simulink model "ES249B_MotAgCorrln"  (R2013b)
settings: Solver=FixedStepDiscrete  SolverMode=SingleTasking  StartTime=0.0  StopTime=1  FixedStep=0.002  RelTol=1e-3
values from neighbouring files (symbols this model uses):
  FLTINJ_MOTAGCORRLN_MOTAGIDPTSIG = DataDict.Constant    [ES249B_MotAgCorrln_DataDict.m]
  HALFREV_MOTREV_U0P16 = DataDict.Constant    [ES249B_MotAgCorrln_DataDict.m]
  MOTAGACORRLNST_CNT_U08 = DataDict.Constant    [ES249B_MotAgCorrln_DataDict.m]
  MotAgAMotAgBCorrln = DataDict.NTC    [ES249B_MotAgCorrln_DataDict.m]
  MOTAGBCORRLNST_CNT_U08 = DataDict.Constant    [ES249B_MotAgCorrln_DataDict.m]
  MOTAGCORRLNERRTHD_MOTREVELEC_U0P16 = DataDict.Constant    [ES249B_MotAgCorrln_DataDict.m]
  MOTAGCORRLNNTCFAILSTEP_CNT_U16 = DataDict.Constant    [ES249B_MotAgCorrln_DataDict.m]
  MOTAGCORRLNNTCPASSSTEP_CNT_U16 = DataDict.Constant    [ES249B_MotAgCorrln_DataDict.m]
  MOTAGMAXSTALLCNTR_CNT_U08 = DataDict.Constant    [ES249B_MotAgCorrln_DataDict.m]
  MotAgMeclCorrlnSt = DataDict.OpSignal    [ES249B_MotAgCorrln_DataDict.m]
  MotAgMeclIdptSig = DataDict.OpSignal    [ES249B_MotAgCorrln_DataDict.m]
  SysGlbPrmMotPoleCnt = DataDict.ImprtdCal    [ES249B_MotAgCorrln_DataDict.m]
undefined symbols (not defined in the file or in its folder): NtcSts1, sigbuilder_block, SigQlfr1
libraries: simulink x5
(part 1 of 2)
settings Model: Creator=pz79n7  LastModifiedBy=FZG88Y
settings SolverCC: AutoInsertRateTranBlk=on  InsertRTBMode=Always
settings DataIOCC: LimitDataPoints=off  SaveFormat=Structure  ReturnWorkspaceOutputs=on
settings OptimizationCC: BlockReduction=off  InlineParams=on  ZeroExternalMemoryAtStartup=off  ZeroInternalMemoryAtStartup=off  OptimizeModelRefInitCode=on  LifeSpan=1
settings DebuggingCC: SignalInfNanChecking=error  SignalRangeChecking=warning  UnderspecifiedInitializationDetection=Simplified  SolverPrmCheckMsg=error  InheritedTsInSrcMsg=error  DiscreteInheritContinuousMsg=error  SingleTaskRateTransMsg=error  TasksWithSamePriorityMsg=error  SigSpecEnsureSampleTimeMsg=error  CheckMatrixSingularityMsg=error  ParameterUnderflowMsg=error  ParameterPrecisionLossMsg=error  ParameterTunabilityLossMsg=error  FixptConstUnderflowMsg=warning  FixptConstOverflowMsg=warning  VectorMatrixConversionMsg=error  SignalLabelMismatchMsg=error  UnconnectedInputMsg=error  UnconnectedOutputMsg=error  UnconnectedLineMsg=error  SFcnCompatibilityMsg=error  UniqueDataStoreMsg=warning  BusObjectLabelMismatch=error  RootOutportRequireBusObject=error  AssertControl=DisableAll  ModelReferenceIOMsg=error  ModelReferenceVersionMismatchMessage=warning  ModelReferenceIOMismatchMessage=error  ModelReferenceCSMismatchMessage=warning  ModelReferenceDataLoggingMessage=error  StateNameClashWarn=warning  StrictBusMsg=ErrorOnBusTreatedAsVector  NonBusSignalsTreatedAsBus=error  SFUnexpectedBacktrackingDiag=error  SFInvalidInputDataAccessInChartInitDiag=error  SFNoUnconditionalDefaultTransitionDiag=error  SFTransitionOutsideNaturalParentDiag=error  SFUnconditionalTransitionShadowingDiag=error  SFUndirectedBroadcastEventsDiag=error
settings ModelReferenceCC: ModelReferenceNumInstancesAllowed=Single
settings RTWCC: SystemTargetFile=autosar.tlc  GenCodeOnly=on  TemplateMakefile=ert_default_tmf  Description=AUTOSAR  GenerateReport=on  ProcessScript=autosar_make_rtw_hook  LaunchReport=on
settings CodeAppCC: GenerateComments=off  IgnoreCustomStorageClasses=off  CustomSymbolStrType=$N$R$M  CustomSymbolStrBlkIO=$N$M  SimulinkBlockComments=off
settings STFCustomTargetCC: ParMdlRefBuildCompliant=on  CompOptLevelCompliant=on  IncludeMdlTerminateFcn=off  CombineOutputUpdateFcns=on  SuppressErrorStatus=on  ERTFirstTimeCompliant=on  ERTCustomFileBanners=on  SupportNonFinite=off  SupportComplex=off  SupportContinuousTime=off  SupportNonInlinedSFcns=off  MATLABClassNameForMDSCustomization=Simulink.SoftwareTarget.ERTCustomization  AutosarCompliant=on  GRTInterface=off  SystemTargetFile=autosar.tlc
settings ERTTargetCC: CodeReplacementLibrary=ANSI_C  ConcurrentExecutionCompliant=off  IncludeMdlTerminateFcn=off  SuppressErrorStatus=on  SupportNonFinite=off  SupportComplex=off  ModelStepFunctionPrototypeControlCompliant=off  CPPClassGenCompliant=off  AutosarCompliant=on  InlinedParameterPlacement=NonHierarchical  ERTCustomFileTemplate=example_file_process.tlc  EnableUserReplacementTypes=on

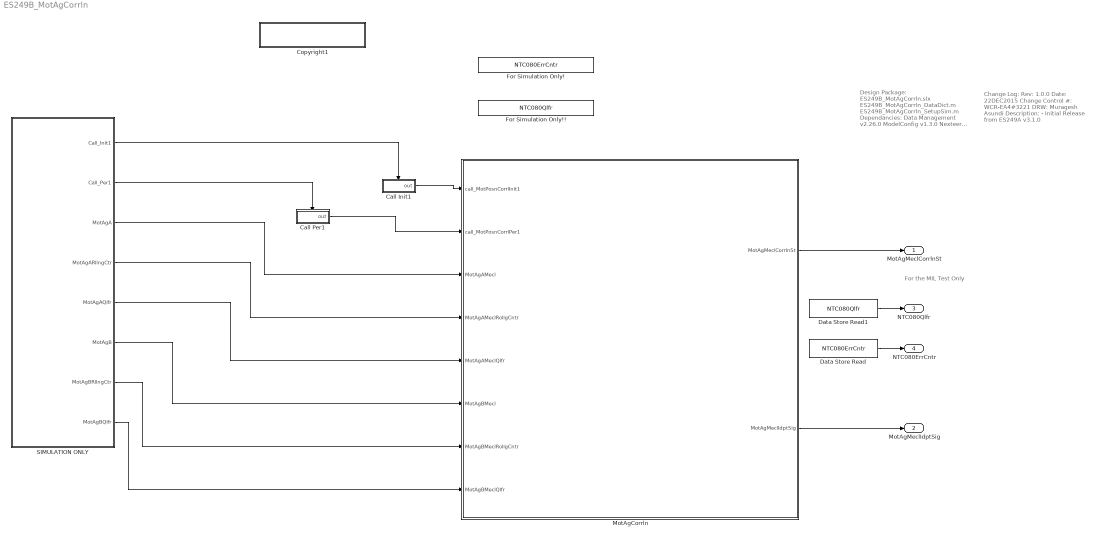
== system ES249B_MotAgCorrln ==
  note: Change Log:
      |
      | Rev: 1.0.0
      | Date: 22DEC2015
      | Change Control #: WCR-EA4#3221
      | DRW: Muragesh Asundi
      | Description:
      | - Initial Release from ES249A v3.1.0
  note: Design Package:
      | ES249B_MotAgCorrln.slx
      | ES249B_MotAgCorrln_DataDict.m
      | ES249B_MotAgCorrln_SetupSim.m
      |
      | Dependancies:
      |    Data Management v2.26.0
      |    ModelConfig v1.3.0
      |    Nexteer Utilities v4.5.0
      |    Tools v1.9.0
      |
      | Requirement: 1.0
  note: For the MIL Test Only
  Call Init1 : Subsystem  TreatAsAtomicUnit=on
  Call Per1 : Subsystem  TreatAsAtomicUnit=on
  Copyright1 : Subsystem  Description=|  mask(Copyright Information){none=on}
      | Copyright info block.                                               
      |                                                                     
      | Place copyright information at the top of every subsystem in design.
      mask prompts: none "No parameters"
      mask help: Place copyright information at the top of every subsystem in design.
      mask Display:
      | NxtrConf = 'Nexteer Confidential';
      | 
      | sys = bdroot; %handle for the current model ("system")
      | first = get_param(sys,'Created');
      | if(isempty(first))
      |     first = datestr(now,'yyyy');
      | else
      |     first = first(end-3:end);  %year is last four digits
      | end
      | 
      | last = get_param(sys,'LastModifiedDate');
      | if isempty(last)
      |     last = datestr(now,'yyyy');
      | else
      |     last = last(end-3:end);
      | end
      | 
      | if strcmp(first,last)
      |     fprintf('%s\nCopyright  %s Nexteer',NxtrConf,first);
      | else
      |     fprintf('%s\n%s%s-%s Nexteer',NxtrConf,char(169),first,last);
      | end
  Data Store Read : DataStoreRead  DataStoreName=NTC080ErrCntr  SampleTime=0.002
  Data Store Read1 : DataStoreRead  DataStoreName=NTC080Qlfr  SampleTime=0.002
  For Simulation Only! : DataStoreMemory  DataStoreName=NTC080ErrCntr
  For Simulation Only!! : DataStoreMemory  DataStoreName=NTC080Qlfr
  MotAgCorrln : Subsystem
  SIMULATION ONLY : Subsystem
  MotAgMeclCorrlnSt : Outport  RequirementInfo={} %GIDa_d8739ec6_a18f_4415_a443_47ea44f287a3
  MotAgMeclIdptSig : Outport  RequirementInfo={} %GIDa_85b325d8_f6bf_41e3_b16b_50e782c8add7  Port=2
  NTC080Qlfr : Outport  RequirementInfo={} %GIDa_3e943792_cbbb_4e5d_9230_63e142ecdc6f  Port=3
  NTC080ErrCntr : Outport  RequirementInfo={} %GIDa_f9c3ca75_2980_486f_8311_d7072cc6ecd3  Port=4
  wires:
  Call Per1/1(out) -> MotAgCorrln/2(call_MotPosnCorrlPer1)
  MotAgCorrln/1(MotAgMeclCorrlnSt) -> MotAgMeclCorrlnSt/1
  MotAgCorrln/2(MotAgMeclIdptSig) -> MotAgMeclIdptSig/1
  SIMULATION ONLY/3(MotAgA) -> MotAgCorrln/3(MotAgAMecl)
  SIMULATION ONLY/4(MotAgARllngCtr) -> MotAgCorrln/4(MotAgAMeclRollgCntr)
  SIMULATION ONLY/5(MotAgAQlfr) -> MotAgCorrln/5(MotAgAMeclQlfr)
  Call Init1/1(out) -> MotAgCorrln/1(call_MotPosnCorrlInit1)
  SIMULATION ONLY/1(Call_Init1) -> Call Init1/Enable
  SIMULATION ONLY/2(Call_Per1) -> Call Per1/Enable
  SIMULATION ONLY/8(MotAgBQlfr) -> MotAgCorrln/8(MotAgBMeclQlfr)
  SIMULATION ONLY/6(MotAgB) -> MotAgCorrln/6(MotAgBMecl)
  SIMULATION ONLY/7(MotAgBRllngCtr) -> MotAgCorrln/7(MotAgBMeclRollgCntr)
  Data Store Read1/1 -> NTC080Qlfr/1
  Data Store Read/1 -> NTC080ErrCntr/1

== system ES249B_MotAgCorrln/Call Init1 ==
  Enable : EnablePort
  Function Call Trigger : simulink/Ports & Subsystems/Function-Call Generator  RequirementInfo={} %GIDa_ff755a2e_49d1_45f7_8591_3ce0ef475338  sample_time=0  numberOfIterations=1
  out : Outport
  wires:
  Function Call Trigger/1 -> out/1

== system ES249B_MotAgCorrln/Call Per1 ==
  Enable : EnablePort
  Function Call Trigger : simulink/Ports & Subsystems/Function-Call Generator  RequirementInfo={} %GIDa_c055ea22_668e_465c_aa17_4b0a8dd99bf7  sample_time=0.002  numberOfIterations=1
  out : Outport
  wires:
  Function Call Trigger/1 -> out/1

== system ES249B_MotAgCorrln/Copyright1 ==

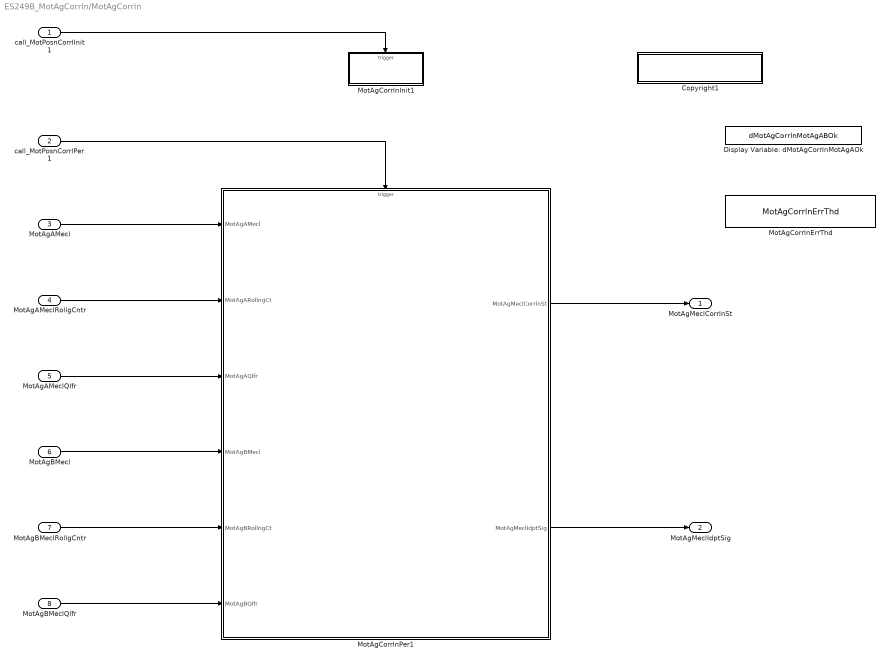
== system ES249B_MotAgCorrln/MotAgCorrln ==
  call_MotPosnCorrlInit1 : Inport  RequirementInfo={} %GIDa_df7b2033_8a98_4878_957d_25acf0131f4b
  call_MotPosnCorrlPer1 : Inport  RequirementInfo={} %GIDa_1551d67e_f818_426a_9cf4_9f4ba82b3f43  Port=2
  MotAgAMecl : Inport  RequirementInfo={'linktype_rmi_doors' '0000cf69 (/E-STEER Core/SubSystem Specifications/Electrical Actuator/Control Module/FDD Module Requirements/EA4/ES249B_MotAgCorrln)' '#ES249B_48' 'true' 'REQ: ES249B_48' '' } %GIDa_ab802314_3944_43a8_9f34_099947b7f787  Port=3
  MotAgAMeclRollgCntr : Inport  RequirementInfo={'linktype_rmi_doors' '0000cf69 (/E-STEER Core/SubSystem Specifications/Electrical Actuator/Control Module/FDD Module Requirements/EA4/ES249B_MotAgCorrln)' '#ES249B_49' 'true' 'REQ: ES249B_49' '' } %GIDa_a38bab73_f7bf_4755_8745_3afc46561306  Port=4
  MotAgAMeclQlfr : Inport  RequirementInfo={'linktype_rmi_doors' '0000cf69 (/E-STEER Core/SubSystem Specifications/Electrical Actuator/Control Module/FDD Module Requirements/EA4/ES249B_MotAgCorrln)' '#ES249B_65' 'true' 'REQ: ES249B_65' '' } %GIDa_033694cf_56a5_4107_96d0_836401cb9721  Port=5
  MotAgBMecl : Inport  RequirementInfo={'linktype_rmi_doors' '0000cf69 (/E-STEER Core/SubSystem Specifications/Electrical Actuator/Control Module/FDD Module Requirements/EA4/ES249B_MotAgCorrln)' '#ES249B_66' 'true' 'REQ: ES249B_66' '' } %GIDa_ed21c9ba_4edb_4b2f_a77a_49cd20ecbf68  Port=6
  MotAgBMeclRollgCntr : Inport  RequirementInfo={'linktype_rmi_doors' '0000cf69 (/E-STEER Core/SubSystem Specifications/Electrical Actuator/Control Module/FDD Module Requirements/EA4/ES249B_MotAgCorrln)' '#ES249B_67' 'true' 'REQ: ES249B_67' '' } %GIDa_6e6bb4b4_2d5c_4f1b_b4e7_5884c06a9259  Port=7
  MotAgBMeclQlfr : Inport  RequirementInfo={'linktype_rmi_doors' '0000cf69 (/E-STEER Core/SubSystem Specifications/Electrical Actuator/Control Module/FDD Module Requirements/EA4/ES249B_MotAgCorrln)' '#ES249B_68' 'true' 'REQ: ES249B_68' '' } %GIDa_842dc15f_0b28_4c0e_80ed_768af48a7cab  Port=8
  Copyright1 : Subsystem  Description=|  RequirementInfo={} %GIDa_dd7bc4e6_4adb_4397_9a47_107977c533a5  mask(Copyright Information){none=on}
      | Copyright info block.                                               
      |                                                                     
      | Place copyright information at the top of every subsystem in design.
      mask prompts: none "No parameters"
      mask help: Place copyright information at the top of every subsystem in design.
      mask Display:
      | NxtrConf = 'Nexteer Confidential';
      | 
      | sys = bdroot; %handle for the current model ("system")
      | first = get_param(sys,'Created');
      | if(isempty(first))
      |     first = datestr(now,'yyyy');
      | else
      |     first = first(end-3:end);  %year is last four digits
      | end
      | 
      | last = get_param(sys,'LastModifiedDate');
      | if isempty(last)
      |     last = datestr(now,'yyyy');
      | else
      |     last = last(end-3:end);
      | end
      | 
      | if strcmp(first,last)
      |     fprintf('%s\nCopyright  %s Nexteer',NxtrConf,first);
      | else
      |     fprintf('%s\n%s%s-%s Nexteer',NxtrConf,char(169),first,last);
      | end
  Display Variable: dMotAgCorrlnMotAgAOk : DataStoreMemory  DataStoreName=dMotAgCorrlnMotAgABOk  StateMustResolveToSignalObject=on
  MotAgCorrlnErrThd : DataStoreMemory  Priority=0  DataStoreName=MotAgCorrlnErrThd  StateMustResolveToSignalObject=on
  MotAgCorrlnInit1 : Subsystem  TreatAsAtomicUnit=on
  MotAgCorrlnPer1 : Subsystem  RequirementInfo={} %GIDa_e8c7526b_9849_4008_8b1a_56f97ffa1c8d  TreatAsAtomicUnit=on
  MotAgMeclCorrlnSt : Outport  RequirementInfo={'linktype_rmi_doors' '0000cf69 (/E-STEER Core/SubSystem Specifications/Electrical Actuator/Control Module/FDD Module Requirements/EA4/ES249B_MotAgCorrln)' '#ES249B_51' 'true' 'REQ: ES249B_51' '' } %GIDa_ae509c2f_e3de_4035_9028_020cbec86e82
  MotAgMeclIdptSig : Outport  RequirementInfo={'linktype_rmi_doors' '0000cf69 (/E-STEER Core/SubSystem Specifications/Electrical Actuator/Control Module/FDD Module Requirements/EA4/ES249B_MotAgCorrln)' '#ES249B_52' 'true' 'REQ: ES249B_52' '' } %GIDa_df68f2b0_a0f0_444f_88a1_35645a7edbac  Port=2
  wires:
  call_MotPosnCorrlPer1/1 -> MotAgCorrlnPer1/Trigger
  MotAgCorrlnPer1/2(MotAgMeclIdptSig) -> MotAgMeclIdptSig/1
  MotAgCorrlnPer1/1(MotAgMeclCorrlnSt) -> MotAgMeclCorrlnSt/1
  MotAgAMecl/1 -> MotAgCorrlnPer1/1(MotAgAMecl)
  MotAgAMeclRollgCntr/1 -> MotAgCorrlnPer1/2(MotAgARollngCt)
  MotAgAMeclQlfr/1 -> MotAgCorrlnPer1/3(MotAgAQlfr)
  MotAgBMecl/1 -> MotAgCorrlnPer1/4(MotAgBMecl)
  MotAgBMeclRollgCntr/1 -> MotAgCorrlnPer1/5(MotAgBRollngCt)
  MotAgBMeclQlfr/1 -> MotAgCorrlnPer1/6(MotAgBQlfr)
  call_MotPosnCorrlInit1/1 -> MotAgCorrlnInit1/Trigger

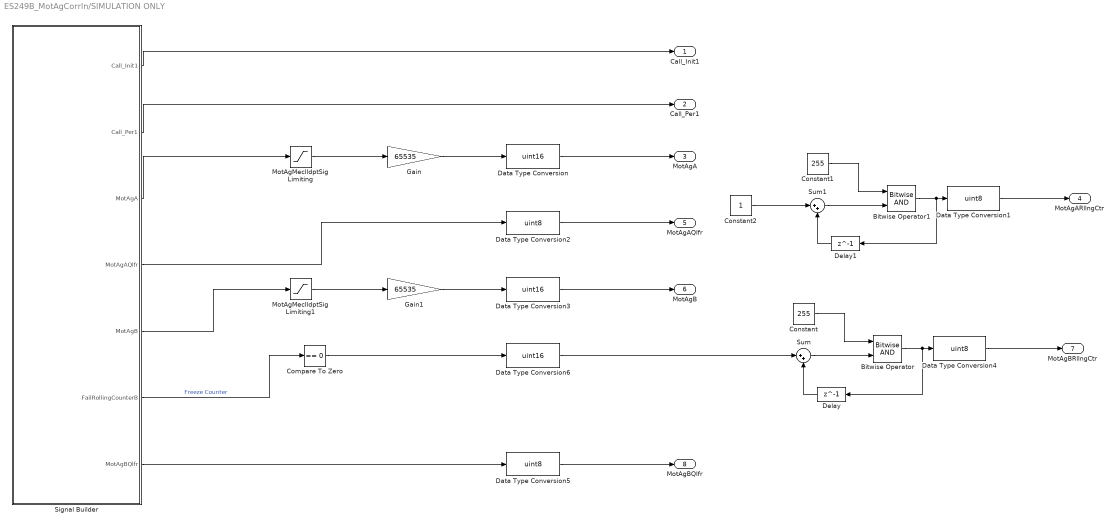
== system ES249B_MotAgCorrln/SIMULATION ONLY ==
  Bitwise Operator : simulink/Logic and Bit Operations/Bitwise Operator  logicop=AND  UseBitMask=off  NumInputPorts=2  BitMask=bin2dec('11011001')  BitMaskRealWorld=Stored Integer
  Bitwise Operator1 : simulink/Logic and Bit Operations/Bitwise Operator  logicop=AND  UseBitMask=off  NumInputPorts=2  BitMask=bin2dec('11011001')  BitMaskRealWorld=Stored Integer
  Compare To Zero : simulink/Logic and Bit Operations/Compare To Zero  relop===  OutDataTypeStr=boolean
  Constant : Constant  Value=255  OutDataTypeStr=uint16
  Constant1 : Constant  Value=255  OutDataTypeStr=uint16
  Constant2 : Constant  OutDataTypeStr=uint16
  Data Type Conversion : DataTypeConversion  OutDataTypeStr=uint16
  Data Type Conversion{1..2,4..5} (4 alike) : DataTypeConversion  OutDataTypeStr=uint8
  Data Type Conversion3 : DataTypeConversion  OutDataTypeStr=uint16
  Data Type Conversion6 : DataTypeConversion  OutDataTypeStr=uint16
  Delay : Delay  DelayLength=1  InitialCondition=0  SampleTime=0.002
  Delay1 : Delay  DelayLength=1  InitialCondition=0  SampleTime=0.002
  Gain : Gain  Gain=65535
  Gain1 : Gain  Gain=65535
  MotAgMeclIdptSig Limiting : Saturate  UpperLimit=1  LowerLimit=0
  MotAgMeclIdptSig Limiting1 : Saturate  UpperLimit=MotAgMeclIdptSig.EngMax  LowerLimit=MotAgMeclIdptSig.EngMin
  Signal Builder : Subsystem  Tag=STV Subsys  LoadFcn=sigbuilder_block('load');  StartFcn=sigbuilder_block('start');  StopFcn=sigbuilder_block('stop');  ClipboardFcn=sigbuilder_block('clipboard');  mask(Sigbuilder block){}
      mask help: Simulink:masks:SigbuilderBlock_MD
      mask init:
      | if ~strcmp(get_param(bdroot(gcbh),'SimulationStatus'),'stopped') tuvar = sigbuilder_block('maskInit'); end
      settings: CopyFcn=sigbuilder_block('copy');  DeleteFcn=sigbuilder_block('delete');  ModelCloseFcn=sigbuilder_block('modelClose');  PreSaveFcn=sigbuilder_block('preSave');  PauseFcn=sigbuilder_block('pause');  ContinueFcn=sigbuilder_block('continue');  NameChangeFcn=sigbuilder_block('namechange');  OpenFcn=sigbuilder_block('open',[6 6 1012.5 507 ]);  CloseFcn=sigbuilder_block('close');
      mask Display: plot(0, 0, 100, 100,[2, 2, 32, 32, 2], [68, 8, 8, 68, 68],[32, 2], [38, 38], [32, 19, 2],[53, 60, 44], [32, 17, 17, 2],[16, 16, 31, 31]);txt = getActiveGroup(gcbh);text(2, 100, txt,'verticalAlignment', 'top');
  Sum : Sum  Inputs=|++
  Sum1 : Sum  Inputs=|++
  Call_Init1 : Outport
  Call_Per1 : Outport  Port=2
  MotAgA : Outport  Port=3
  MotAgARllngCtr : Outport  Port=4
  MotAgAQlfr : Outport  Port=5
  MotAgB : Outport  Port=6
  MotAgBRllngCtr : Outport  Port=7
  MotAgBQlfr : Outport  Port=8
  wires:
  Signal Builder/3(MotAgA) -> MotAgMeclIdptSig Limiting/1
  Signal Builder/4(MotAgAQlfr) -> Data Type Conversion2/1
  Signal Builder/5(MotAgB) -> MotAgMeclIdptSig Limiting1/1
  Gain/1 -> Data Type Conversion/1
  Gain1/1 -> Data Type Conversion3/1
  Data Type Conversion4/1 -> MotAgBRllngCtr/1
  Data Type Conversion/1 -> MotAgA/1
  Data Type Conversion2/1 -> MotAgAQlfr/1
  Signal Builder/6(FailRollingCounterB) -> Compare To Zero/1  "Freeze Counter"
  Data Type Conversion3/1 -> MotAgB/1
  MotAgMeclIdptSig Limiting/1 -> Gain/1
  MotAgMeclIdptSig Limiting1/1 -> Gain1/1
  Compare To Zero/1 -> Data Type Conversion6/1
  Data Type Conversion6/1 -> Sum/1
  Delay/1 -> Sum/2
  Constant/1 -> Bitwise Operator/1
  Sum/1 -> Bitwise Operator/2
  Bitwise Operator/1 -> Delay/1, Data Type Conversion4/1
  Delay1/1 -> Sum1/2
  Constant1/1 -> Bitwise Operator1/1
  Sum1/1 -> Bitwise Operator1/2
  Bitwise Operator1/1 -> Data Type Conversion1/1, Delay1/1
  Data Type Conversion1/1 -> MotAgARllngCtr/1
  Constant2/1 -> Sum1/1
  Signal Builder/1(Call_Init1) -> Call_Init1/1
  Signal Builder/2(Call_Per1) -> Call_Per1/1
  Signal Builder/7(MotAgBQlfr) -> Data Type Conversion5/1
  Data Type Conversion5/1 -> MotAgBQlfr/1

== system ES249B_MotAgCorrln/MotAgCorrln/Copyright1 ==

== system ES249B_MotAgCorrln/MotAgCorrln/MotAgCorrlnInit1 ==
  function : TriggerPort  TriggerType=function-call
  Compute Error Threshold : Subsystem  TreatAsAtomicUnit=on
  Copyright1 : Subsystem  Description=|  RequirementInfo={} %GIDa_76facc10_fa9f_4b93_b759_726016e2f92e  mask(Copyright Information){none=on}
      | Copyright info block.                                               
      |                                                                     
      | Place copyright information at the top of every subsystem in design.
      mask prompts: none "No parameters"
      mask help: Place copyright information at the top of every subsystem in design.
      mask Display:
      | NxtrConf = 'Nexteer Confidential';
      | 
      | sys = bdroot; %handle for the current model ("system")
      | first = get_param(sys,'Created');
      | if(isempty(first))
      |     first = datestr(now,'yyyy');
      | else
      |     first = first(end-3:end);  %year is last four digits
      | end
      | 
      | last = get_param(sys,'LastModifiedDate');
      | if isempty(last)
      |     last = datestr(now,'yyyy');
      | else
      |     last = last(end-3:end);
      | end
      | 
      | if strcmp(first,last)
      |     fprintf('%s\nCopyright  %s Nexteer',NxtrConf,first);
      | else
      |     fprintf('%s\n%s%s-%s Nexteer',NxtrConf,char(169),first,last);
      | end

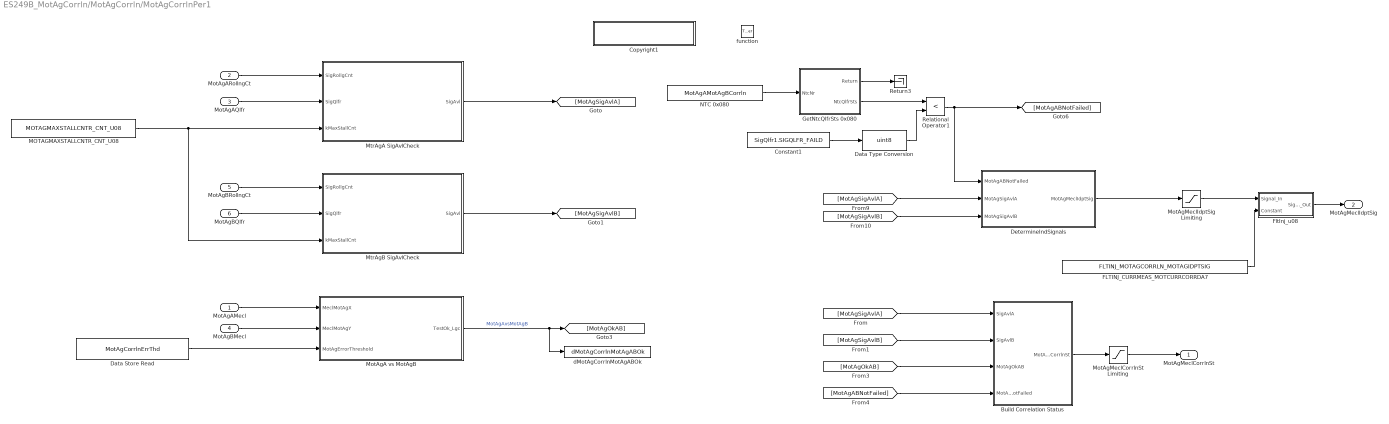
== system ES249B_MotAgCorrln/MotAgCorrln/MotAgCorrlnPer1 ==
  MotAgAMecl : Inport  RequirementInfo={} %GIDa_0d510189_b4be_492d_be7e_b68d691b2df9
  MotAgARollngCt : Inport  RequirementInfo={} %GIDa_517e33a2_5a75_4f61_8f0f_573ac68cba90  Port=2
  MotAgAQlfr : Inport  RequirementInfo={} %GIDa_72867f98_7693_466f_aee4_0d6354195f1e  Port=3
  MotAgBMecl : Inport  RequirementInfo={} %GIDa_cfbccf8f_533e_4f37_986a_e6dac4ce98be  Port=4
  MotAgBRollngCt : Inport  RequirementInfo={} %GIDa_0bfa8ef6_2836_4615_abbf_8888cb320397  Port=5
  MotAgBQlfr : Inport  RequirementInfo={} %GIDa_efd6d5fa_412f_4474_a057_389b850e160a  Port=6
  function : TriggerPort  RequirementInfo={} %GIDa_31db59e0_dbe3_46c8_b533_8d5601b81075  TriggerType=function-call
  Build Correlation Status : Subsystem  RequirementInfo={'linktype_rmi_doors' '0000cf69 (/E-STEER Core/SubSystem Specifications/Electrical Actuator/Control Module/FDD Module Requirements/EA4/ES249B_MotAgCorrln)' '#ES249B_90' 'true' 'REQ: ES249B_90' '' ; 'linktype_rmi_doors' '0000cf69 (/E-STEER Core/SubSystem Specifications/Electrical Actuator/Control Module/FDD Module Requirements/EA4/ES249B_MotAgCorrln)' '#ES249B_91' 'true' 'REQ: ES249B_91' '' ; 'linktype_rmi_doors' '0000cf69 (/E-STEER Core/SubSystem Specifications/Electrical Actuator/Control Module/FDD Module Requirements/EA4/ES249B_MotAgCorrln)' '#ES249B_93' 'true' 'REQ: ES249B_93' '' } %GIDa_4418b42c_053d_4239_93e1_04840cd9c1ab
  Constant1 : Constant  Value=SigQlfr1.SIGQLFR_FAILD  OutDataTypeStr=Enum: SigQlfr1
      settings: AttributesFormatString=%<OutDataTypeStr>
  Copyright1 : Subsystem  Description=|  RequirementInfo={} %GIDa_7b6edb4a_3f39_48e0_befb_44ef32e9295a  mask(Copyright Information){none=on}
      | Copyright info block.                                               
      |                                                                     
      | Place copyright information at the top of every subsystem in design.
      mask prompts: none "No parameters"
      mask help: Place copyright information at the top of every subsystem in design.
      mask Display:
      | NxtrConf = 'Nexteer Confidential';
      | 
      | sys = bdroot; %handle for the current model ("system")
      | first = get_param(sys,'Created');
      | if(isempty(first))
      |     first = datestr(now,'yyyy');
      | else
      |     first = first(end-3:end);  %year is last four digits
      | end
      | 
      | last = get_param(sys,'LastModifiedDate');
      | if isempty(last)
      |     last = datestr(now,'yyyy');
      | else
      |     last = last(end-3:end);
      | end
      | 
      | if strcmp(first,last)
      |     fprintf('%s\nCopyright  %s Nexteer',NxtrConf,first);
      | else
      |     fprintf('%s\n%s%s-%s Nexteer',NxtrConf,char(169),first,last);
      | end
  Data Store Read : DataStoreRead  DataStoreName=MotAgCorrlnErrThd
  Data Type Conversion : DataTypeConversion  OutDataTypeStr=uint8
  DetermineIndSignals : Subsystem  RequirementInfo={'linktype_rmi_doors' '0000cf69 (/E-STEER Core/SubSystem Specifications/Electrical Actuator/Control Module/FDD Module Requirements/EA4/ES249B_MotAgCorrln)' '#ES249B_96' 'true' 'REQ: ES249B_96' '' ; 'linktype_rmi_doors' '0000cf69 (/E-STEER Core/SubSystem Specifications/Electrical Actuator/Control Module/FDD Module Requirements/EA4/ES249B_MotAgCorrln)' '#ES249B_101' 'true' 'REQ: ES249B_101' '' } %GIDa_0b74bb57_7518_455c_ba25_57387d767c3e
  FLTINJ_CURRMEAS_MOTCURRCORRDA7 : Constant  Value=FLTINJ_MOTAGCORRLN_MOTAGIDPTSIG
  "FltInj_u08 " : Subsystem  RequirementInfo={'linktype_rmi_doors' '0000cf69 (/E-STEER Core/SubSystem Specifications/Electrical Actuator/Control Module/FDD Module Requirements/EA4/ES249B_MotAgCorrln)' '#ES249B_106' 'true' 'REQ: ES249B_106' '' } %GIDa_071c3215_62aa_4359_8caf_75f09dd6c30e  TreatAsAtomicUnit=on  VariantControl=FltInj_sim  mask(Fault_Injection){}
      mask help: Fault Injection is a simulation only block for EA3 programs.
  "GetNtcQlfrSts 0x080 " : Subsystem  RequirementInfo={'linktype_rmi_doors' '0000cf69 (/E-STEER Core/SubSystem Specifications/Electrical Actuator/Control Module/FDD Module Requirements/EA4/ES249B_MotAgCorrln)' '#ES249B_91' 'true' 'REQ: ES249B_91' '' ; 'linktype_rmi_doors' '0000cf69 (/E-STEER Core/SubSystem Specifications/Electrical Actuator/Control Module/FDD Module Requirements/EA4/ES249B_MotAgCorrln)' '#ES249B_93' 'true' 'REQ: ES249B_93' '' } %GIDa_cf545445_441a_46fe_b236_5e2b4963b333
  MOTAGMAXSTALLCNTR_CNT_U08 : Constant  RequirementInfo={} %GIDa_608cf4f3_c4d9_4650_bf98_959cd5939cb0  Value=MOTAGMAXSTALLCNTR_CNT_U08
  MotAgA vs MotAgB : Subsystem  RequirementInfo={'linktype_rmi_doors' '0000cf69 (/E-STEER Core/SubSystem Specifications/Electrical Actuator/Control Module/FDD Module Requirements/EA4/ES249B_MotAgCorrln)' '#ES249B_25' 'true' 'REQ: ES249B_25' '' ; 'linktype_rmi_doors' '0000cf69 (/E-STEER Core/SubSystem Specifications/Electrical Actuator/Control Module/FDD Module Requirements/EA4/ES249B_MotAgCorrln)' '#ES249B_22' 'true' 'REQ: ES249B_22' '' } %GIDa_09b3f2ca_3360_4937_963b_0a8119aa0d87  TreatAsAtomicUnit=on
  MotAgMeclCorrlnSt Limiting : Saturate  UpperLimit=MotAgMeclCorrlnSt.EngMax  LowerLimit=MotAgMeclCorrlnSt.EngMin
  MotAgMeclIdptSig Limiting : Saturate  UpperLimit=MotAgMeclIdptSig.EngMax  LowerLimit=MotAgMeclIdptSig.EngMin
  MtrAgA SigAvlCheck : Subsystem  RequirementInfo={'linktype_rmi_doors' '0000cf69 (/E-STEER Core/SubSystem Specifications/Electrical Actuator/Control Module/FDD Module Requirements/EA4/ES249B_MotAgCorrln)' '#ES249B_53' 'true' 'REQ: ES249B_53' '' } %GIDa_7d20d3b5_defb_4845_b48d_75bf829e2c25  TreatAsAtomicUnit=on
  MtrAgB SigAvlCheck : Subsystem  RequirementInfo={'linktype_rmi_doors' '0000cf69 (/E-STEER Core/SubSystem Specifications/Electrical Actuator/Control Module/FDD Module Requirements/EA4/ES249B_MotAgCorrln)' '#ES249B_53' 'true' 'REQ: ES249B_53' '' } %GIDa_e439906c_aead_491e_9a6c_f8170eb4d0a5  TreatAsAtomicUnit=on
  NTC 0x080 : Constant  RequirementInfo={} %GIDa_0eea48c0_45e5_4398_a9be_a03239322b48  Value=MotAgAMotAgBCorrln
  Relational Operator1 : RelationalOperator  Operator=<  OutDataTypeStr=boolean
  Return3 : Terminator
      settings: RequirementInfo={} %GIDa_c9e19320_3f8d_4741_896e_f243d7830e4c
  dMotAgCorrlnMotAgABOk : DataStoreWrite  RequirementInfo={} %GIDa_83af0017_845d_42a9_9791_0193bed95843  DataStoreName=dMotAgCorrlnMotAgABOk
  MotAgMeclCorrlnSt : Outport  RequirementInfo={} %GIDa_e94f5450_01bd_4b33_9e8b_f067b81cb070
  MotAgMeclIdptSig : Outport  RequirementInfo={} %GIDa_f44c3d14_99ac_4145_ace9_f5b4313ef171  Port=2  OutDataTypeStr=uint8
  wires:
  MOTAGMAXSTALLCNTR_CNT_U08/1 -> MtrAgB SigAvlCheck/3(kMaxStallCnt), MtrAgA SigAvlCheck/3(kMaxStallCnt)
  MtrAgA SigAvlCheck/1(SigAvl) -> [MotAgSigAvlA]
  MotAgA vs MotAgB/1(TestOk_Lgc) -> dMotAgCorrlnMotAgABOk/1, [MotAgOkAB]  "MotAgAvsMotAgB"
  NTC 0x080/1 -> "GetNtcQlfrSts 0x080 "/1(NtcNr)
  "GetNtcQlfrSts 0x080 "/1(Return) -> Return3/1
  MtrAgB SigAvlCheck/1(SigAvl) -> [MotAgSigAvlB]
  Data Store Read/1 -> MotAgA vs MotAgB/3(MotAgErrorThreshold)
  MotAgMeclCorrlnSt Limiting/1 -> MotAgMeclCorrlnSt/1
  MotAgMeclIdptSig Limiting/1 -> "FltInj_u08 "/1(Signal_In)
  "FltInj_u08 "/1(Signal_Out) -> MotAgMeclIdptSig/1
  FLTINJ_CURRMEAS_MOTCURRCORRDA7/1 -> "FltInj_u08 "/2(Constant)
  MotAgBRollngCt/1 -> MtrAgB SigAvlCheck/1(SigRollgCnt)
  MotAgBQlfr/1 -> MtrAgB SigAvlCheck/2(SigQlfr)
  MotAgAMecl/1 -> MotAgA vs MotAgB/1(MeclMotAgX)
  MotAgBMecl/1 -> MotAgA vs MotAgB/2(MeclMotAgY)
  MotAgARollngCt/1 -> MtrAgA SigAvlCheck/1(SigRollgCnt)
  MotAgAQlfr/1 -> MtrAgA SigAvlCheck/2(SigQlfr)
  [MotAgSigAvlA] -> DetermineIndSignals/2(MotAgSigAvlA)
  [MotAgSigAvlB] -> DetermineIndSignals/3(MotAgSigAvlB)
  "GetNtcQlfrSts 0x080 "/2(NtcQlfrSts) -> Relational Operator1/1
  Relational Operator1/1 -> DetermineIndSignals/1(MotAgABNotFailed), [MotAgABNotFailed]
  DetermineIndSignals/1(MotAgMeclIdptSig) -> MotAgMeclIdptSig Limiting/1
  [MotAgABNotFailed] -> Build Correlation Status/4(MotAgABNotFailed)
  [MotAgOkAB] -> Build Correlation Status/3(MotAgOkAB)
  [MotAgSigAvlA] -> Build Correlation Status/1(SigAvlA)
  [MotAgSigAvlB] -> Build Correlation Status/2(SigAvlB)
  Build Correlation Status/1(MotAgMeclCorrlnSt) -> MotAgMeclCorrlnSt Limiting/1
  Data Type Conversion/1 -> Relational Operator1/2
  Constant1/1 -> Data Type Conversion/1

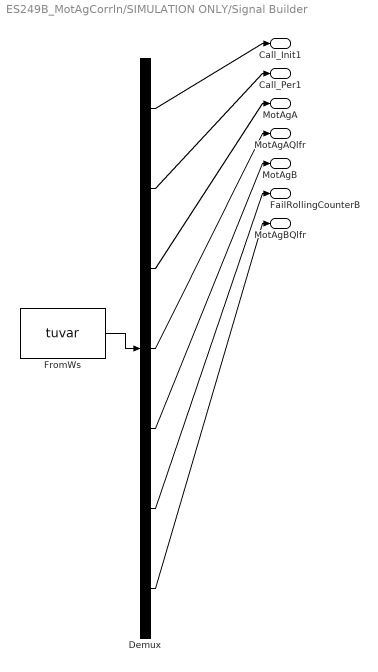
== system ES249B_MotAgCorrln/SIMULATION ONLY/Signal Builder ==
  Demux : Demux  Tag=STV Demux  Outputs=7
  FromWs : FromWorkspace  Tag=STV FromWs  VariableName=tuvar  SampleTime=0
      SigBuilderData=|
      | common.afterFinalStr = 'Extrapolate'
      | common.sampleTime = 0
      | dataSet(1).timeRange = [0 10]
      | dataSet(1).name = 'MotAgAandBFail'
      | dataSet(2).timeRange = [0 10]
      | dataSet(2).name = 'FailAngleB'
      | dataSet(3).timeRange = [0 10]
      | dataSet(3).name = 'MotAgCFails'
      | dataSet(4).timeRange = [0 10]
      | dataSet(4).name = 'QualOnAFails2'
      | dataSet(5).timeRange = [0 10]
      | dataSet(5).name = 'FrozenCounterB'
      | dataSet(6).timeRange = [0 10]
      | dataSet(6).name = 'Rollover of signal misalignment'
      | dataSet(7).timeRange = [0 10]
      | dataSet(7).name = 'Rollover of signal misalignment in opposite direction'
      | dataSet(8).timeRange = [0 10]
      | dataSet(8).name = 'MotAgAandBFail1'
      | sbobj.Groups(1).Name = 'MotAgAandBFail'
      | sbobj.Groups(1).Signals(1).Name = 'Call_Init1'
      | sbobj.Groups(1).Signals(1).XData = [0 10]
      | sbobj.Groups(1).Signals(1).YData = [0 0]
      | sbobj.Groups(1).Signals(2).Name = 'Call_Per1'
      | sbobj.Groups(1).Signals(2).XData = [0 0.002 0.002 10]
      | sbobj.Groups(1).Signals(2).YData = [1 1 0 0]
      | sbobj.Groups(1).Signals(3).Name = 'MotAgA'
      | sbobj.Groups(1).Signals(3).XData = [0 0.020202020202 0.040404040404 0.0606060606061 0.0808080808081 0.10101010101 0.121212121212 0.141414141414 0.161616161616 0.181818181818 0.20202020202 0.222222222222 ... (496 elements, 1x496)]
      | sbobj.Groups(1).Signals(3).YData = [0.5 0.531711959828 0.563296226787 0.59462562218 0.625573993591 0.656016722849 0.68583122783 0.714897456045 0.74309836805 0.770320408728 0.796453964527 0.821393804843 ... (496 elements, 1x496)]
      | sbobj.Groups(1).Signals(4).Name = 'MotAgAQlfr'
      | sbobj.Groups(1).Signals(4).XData = [0 0.305 1 1 3.005 3.005 10]
      | sbobj.Groups(1).Signals(4).YData = [1 1 1 2 1 2 2]
      | sbobj.Groups(1).Signals(5).Name = 'MotAgB'
      | sbobj.Groups(1).Signals(5).XData = [0 0.020202020202 0.040404040404 0.0606060606061 0.0808080808081 0.10101010101 0.121212121212 0.141414141414 0.161616161616 0.181818181818 0.20202020202 0.222222222222 ... (500 elements, 1x500)]
      | sbobj.Groups(1).Signals(5).YData = [0.5 0.531711959828 0.563296226787 0.59462562218 0.625573993591 0.656016722849 0.68583122783 0.714897456045 0.74309836805 0.770320408728 0.796453964527 0.821393804843 ... (500 elements, 1x500)]
      | sbobj.Groups(1).Signals(6).Name = 'FailRollingCounterB'
      | sbobj.Groups(1).Signals(6).XData = [0 0.5 10]
      | sbobj.Groups(1).Signals(6).YData = [0 0 0]
      | sbobj.Groups(1).Signals(7).Name = 'MotAgBQlfr'
      | sbobj.Groups(1).Signals(7).XData = [0 10]
      | sbobj.Groups(1).Signals(7).YData = [1 1]
      | sbobj.Groups(2).Name = 'FailAngleB'
      | sbobj.Groups(2).Signals(1).Name = 'Call_Init1'
      | sbobj.Groups(2).Signals(1).XData = [0 10]
      | sbobj.Groups(2).Signals(1).YData = [0 0]
      | sbobj.Groups(2).Signals(2).Name = 'Call_Per1'
      | sbobj.Groups(2).Signals(2).XData = [0 0.002 0.002 10]
      | sbobj.Groups(2).Signals(2).YData = [1 1 0 0]
      | sbobj.Groups(2).Signals(3).Name = 'MotAgA'
      | sbobj.Groups(2).Signals(3).XData = [0 0.020202020202 0.040404040404 0.0606060606061 0.0808080808081 0.10101010101 0.121212121212 0.141414141414 0.161616161616 0.181818181818 0.20202020202 0.222222222222 ... (496 elements, 1x496)]
      | sbobj.Groups(2).Signals(3).YData = [0.5 0.531711959828 0.563296226787 0.59462562218 0.625573993591 0.656016722849 0.68583122783 0.714897456045 0.74309836805 0.770320408728 0.796453964527 0.821393804843 ... (496 elements, 1x496)]
      | sbobj.Groups(2).Signals(4).Name = 'MotAgAQlfr'
      | sbobj.Groups(2).Signals(4).XData = [0 0.305 1 1 3.005 3.005 10]
      | sbobj.Groups(2).Signals(4).YData = [1 1 1 2 1 2 2]
      | sbobj.Groups(2).Signals(5).Name = 'MotAgB'
      | sbobj.Groups(2).Signals(5).XData = [0 0.020202020202 0.040404040404 0.0606060606061 0.0808080808081 0.10101010101 0.121212121212 0.141414141414 0.161616161616 0.181818181818 0.20202020202 0.222222222222 ... (496 elements, 1x496)]
      | sbobj.Groups(2).Signals(5).YData = [0.5 0.531711959828 0.563296226787 0.59462562218 0.625573993591 0.656016722849 0.68583122783 0.714897456045 0.74309836805 0.770320408728 0.796453964527 0.821393804843 ... (496 elements, 1x496)]
      | sbobj.Groups(2).Signals(6).Name = 'FailRollingCounterB'
      | sbobj.Groups(2).Signals(6).XData = [0 0.5 10]
      | sbobj.Groups(2).Signals(6).YData = [0 0 0]
      | sbobj.Groups(2).Signals(7).Name = 'MotAgBQlfr'
      | sbobj.Groups(2).Signals(7).XData = [0 10]
      | sbobj.Groups(2).Signals(7).YData = [1 1]
      | sbobj.Groups(3).Name = 'MotAgCFails'
      | sbobj.Groups(3).Signals(1).Name = 'Call_Init1'
      | sbobj.Groups(3).Signals(1).XData = [0 10]
      | sbobj.Groups(3).Signals(1).YData = [0 0]
      | sbobj.Groups(3).Signals(2).Name = 'Call_Per1'
      | sbobj.Groups(3).Signals(2).XData = [0 0.002 0.002 10]
      | sbobj.Groups(3).Signals(2).YData = [1 1 0 0]
      | sbobj.Groups(3).Signals(3).Name = 'MotAgA'
      | sbobj.Groups(3).Signals(3).XData = [0 0.020202020202 0.040404040404 0.0606060606061 0.0808080808081 0.10101010101 0.121212121212 0.141414141414 0.161616161616 0.181818181818 0.20202020202 0.222222222222 ... (496 elements, 1x496)]
      | sbobj.Groups(3).Signals(3).YData = [0.5 0.531711959828 0.563296226787 0.59462562218 0.625573993591 0.656016722849 0.68583122783 0.714897456045 0.74309836805 0.770320408728 0.796453964527 0.821393804843 ... (496 elements, 1x496)]
      | sbobj.Groups(3).Signals(4).Name = 'MotAgAQlfr'
      | sbobj.Groups(3).Signals(4).XData = [0 0.305 1 1 3.005 3.005 10]
      | sbobj.Groups(3).Signals(4).YData = [1 1 1 2 1 2 2]
      | sbobj.Groups(3).Signals(5).Name = 'MotAgB'
      | sbobj.Groups(3).Signals(5).XData = [0 0.020202020202 0.040404040404 0.0606060606061 0.0808080808081 0.10101010101 0.121212121212 0.141414141414 0.161616161616 0.181818181818 0.20202020202 0.222222222222 ... (496 elements, 1x496)]
      | sbobj.Groups(3).Signals(5).YData = [0.5 0.531711959828 0.563296226787 0.59462562218 0.625573993591 0.656016722849 0.68583122783 0.714897456045 0.74309836805 0.770320408728 0.796453964527 0.821393804843 ... (496 elements, 1x496)]
      | sbobj.Groups(3).Signals(6).Name = 'FailRollingCounterB'
      | sbobj.Groups(3).Signals(6).XData = [0 0.5 10]
      | sbobj.Groups(3).Signals(6).YData = [0 0 0]
      | sbobj.Groups(3).Signals(7).Name = 'MotAgBQlfr'
      | sbobj.Groups(3).Signals(7).XData = [0 10]
      | sbobj.Groups(3).Signals(7).YData = [1 1]
      | sbobj.Groups(4).Name = 'QualOnAFails2'
      | sbobj.Groups(4).Signals(1).Name = 'Call_Init1'
      | sbobj.Groups(4).Signals(1).XData = [0 10]
      | sbobj.Groups(4).Signals(1).YData = [0 0]
      | sbobj.Groups(4).Signals(2).Name = 'Call_Per1'
      | sbobj.Groups(4).Signals(2).XData = [0 0.002 0.002 10]
      | sbobj.Groups(4).Signals(2).YData = [1 1 0 0]
      | sbobj.Groups(4).Signals(3).Name = 'MotAgA'
      | sbobj.Groups(4).Signals(3).XData = [0 0.020202020202 0.040404040404 0.0606060606061 0.0808080808081 0.10101010101 0.121212121212 0.141414141414 0.161616161616 0.181818181818 0.20202020202 0.222222222222 ... (496 elements, 1x496)]
      | sbobj.Groups(4).Signals(3).YData = [0.5 0.531711959828 0.563296226787 0.59462562218 0.625573993591 0.656016722849 0.68583122783 0.714897456045 0.74309836805 0.770320408728 0.796453964527 0.821393804843 ... (496 elements, 1x496)]
      | sbobj.Groups(4).Signals(4).Name = 'MotAgAQlfr'
      | sbobj.Groups(4).Signals(4).XData = [0 0.305 0.305 1 3.005 3.005 10]
      | sbobj.Groups(4).Signals(4).YData = [1 1 2 2 1 2 2]
      | sbobj.Groups(4).Signals(5).Name = 'MotAgB'
      | sbobj.Groups(4).Signals(5).XData = [0 0.020202020202 0.040404040404 0.0606060606061 0.0808080808081 0.10101010101 0.121212121212 0.141414141414 0.161616161616 0.181818181818 0.20202020202 0.222222222222 ... (496 elements, 1x496)]
      | sbobj.Groups(4).Signals(5).YData = [0.5 0.531711959828 0.563296226787 0.59462562218 0.625573993591 0.656016722849 0.68583122783 0.714897456045 0.74309836805 0.770320408728 0.796453964527 0.821393804843 ... (496 elements, 1x496)]
      | sbobj.Groups(4).Signals(6).Name = 'FailRollingCounterB'
      | sbobj.Groups(4).Signals(6).XData = [0 0.5 10]
      | sbobj.Groups(4).Signals(6).YData = [0 0 0]
      | sbobj.Groups(4).Signals(7).Name = 'MotAgBQlfr'
      | sbobj.Groups(4).Signals(7).XData = [0 10]
      | sbobj.Groups(4).Signals(7).YData = [1 1]
      | sbobj.Groups(5).Name = 'FrozenCounterB'
      | sbobj.Groups(5).Signals(1).Name = 'Call_Init1'
      | sbobj.Groups(5).Signals(1).XData = [0 10]
      | sbobj.Groups(5).Signals(1).YData = [0 0]
      | sbobj.Groups(5).Signals(2).Name = 'Call_Per1'
      | sbobj.Groups(5).Signals(2).XData = [0 0.002 0.002 10]
      | sbobj.Groups(5).Signals(2).YData = [1 1 0 0]
      | sbobj.Groups(5).Signals(3).Name = 'MotAgA'
      | sbobj.Groups(5).Signals(3).XData = [0 0.020202020202 0.040404040404 0.0606060606061 0.0808080808081 0.10101010101 0.121212121212 0.141414141414 0.161616161616 0.181818181818 0.20202020202 0.222222222222 ... (496 elements, 1x496)]
      | sbobj.Groups(5).Signals(3).YData = [0.5 0.531711959828 0.563296226787 0.59462562218 0.625573993591 0.656016722849 0.68583122783 0.714897456045 0.74309836805 0.770320408728 0.796453964527 0.821393804843 ... (496 elements, 1x496)]
      | sbobj.Groups(5).Signals(4).Name = 'MotAgAQlfr'
      | sbobj.Groups(5).Signals(4).XData = [0 0.305 1 1 3.005 3.005 10]
      | sbobj.Groups(5).Signals(4).YData = [1 1 1 2 1 2 2]
      | sbobj.Groups(5).Signals(5).Name = 'MotAgB'
      | sbobj.Groups(5).Signals(5).XData = [0 0.020202020202 0.040404040404 0.0606060606061 0.0808080808081 0.10101010101 0.121212121212 0.141414141414 0.161616161616 0.181818181818 0.20202020202 0.222222222222 ... (496 elements, 1x496)]
      | sbobj.Groups(5).Signals(5).YData = [0.5 0.531711959828 0.563296226787 0.59462562218 0.625573993591 0.656016722849 0.68583122783 0.714897456045 0.74309836805 0.770320408728 0.796453964527 0.821393804843 ... (496 elements, 1x496)]
      | sbobj.Groups(5).Signals(6).Name = 'FailRollingCounterB'
      | sbobj.Groups(5).Signals(6).XData = [0 0.138 0.138 0.4 0.4 10]
      | sbobj.Groups(5).Signals(6).YData = [0 0 1 1 0 1]
      | sbobj.Groups(5).Signals(7).Name = 'MotAgBQlfr'
      | sbobj.Groups(5).Signals(7).XData = [0 10]
      | sbobj.Groups(5).Signals(7).YData = [1 1]
      | sbobj.Groups(6).Name = 'Rollover of signal misalignment'
      | sbobj.Groups(6).Signals(1).Name = 'Call_Init1'
      | sbobj.Groups(6).Signals(1).XData = [0 0.002 0.002 10]
      | sbobj.Groups(6).Signals(1).YData = [1 1 0 0]
      | sbobj.Groups(6).Signals(2).Name = 'Call_Per1'
      | sbobj.Groups(6).Signals(2).XData = [0 0.004 0.004 10]
      | sbobj.Groups(6).Signals(2).YData = [0 0 1 1]
      | sbobj.Groups(6).Signals(3).Name = 'MotAgA'
      | sbobj.Groups(6).Signals(3).XData = [0 0.4 0.4 0.7 0.7 10]
      | sbobj.Groups(6).Signals(3).YData = [0 1 0 1 0 0]
      | sbobj.Groups(6).Signals(4).Name = 'MotAgAQlfr'
      | sbobj.Groups(6).Signals(4).XData = [0 0.305 1 1 3.005 3.005 10]
      | sbobj.Groups(6).Signals(4).YData = [1 1 1 2 1 2 2]
      | sbobj.Groups(6).Signals(5).Name = 'MotAgB'
      | sbobj.Groups(6).Signals(5).XData = [0 0.392 0.392 0.707 0.707 10]
      | sbobj.Groups(6).Signals(5).YData = [0 1 0 1 0 0]
      | sbobj.Groups(6).Signals(6).Name = 'FailRollingCounterB'
      | sbobj.Groups(6).Signals(6).XData = [0 0.138 0.4 10]
      | sbobj.Groups(6).Signals(6).YData = [0 0 0 1]
      | sbobj.Groups(6).Signals(7).Name = 'MotAgBQlfr'
      | sbobj.Groups(6).Signals(7).XData = [0 10]
      | sbobj.Groups(6).Signals(7).YData = [1 1]
      | sbobj.Groups(7).Name = 'Rollover of signal misalignment in opposite direction'
      | sbobj.Groups(7).Signals(1).Name = 'Call_Init1'
      | sbobj.Groups(7).Signals(1).XData = [0 0.002 0.002 10]
      | sbobj.Groups(7).Signals(1).YData = [1 1 0 0]
      | sbobj.Groups(7).Signals(2).Name = 'Call_Per1'
      | sbobj.Groups(7).Signals(2).XData = [0 0.004 0.004 10]
      | sbobj.Groups(7).Signals(2).YData = [0 0 1 1]
      | sbobj.Groups(7).Signals(3).Name = 'MotAgA'
      | sbobj.Groups(7).Signals(3).XData = [0 0.4 0.4 0.7 0.7 1 10]
      | sbobj.Groups(7).Signals(3).YData = [1 0 1 0 1 0 0]
      | sbobj.Groups(7).Signals(4).Name = 'MotAgAQlfr'
      | sbobj.Groups(7).Signals(4).XData = [0 0.305 1 1 3.005 3.005 10]
      | sbobj.Groups(7).Signals(4).YData = [1 1 1 2 1 2 2]
      | sbobj.Groups(7).Signals(5).Name = 'MotAgB'
      | sbobj.Groups(7).Signals(5).XData = [0 0.392 0.392 0.707 0.707 1 10]
      | sbobj.Groups(7).Signals(5).YData = [1 0 1 0 1 0 0]
      | sbobj.Groups(7).Signals(6).Name = 'FailRollingCounterB'
      | sbobj.Groups(7).Signals(6).XData = [0 0.138 0.4 10]
      | sbobj.Groups(7).Signals(6).YData = [0 0 0 1]
      | sbobj.Groups(7).Signals(7).Name = 'MotAgBQlfr'
      | sbobj.Groups(7).Signals(7).XData = [0 10]
      | sbobj.Groups(7).Signals(7).YData = [1 1]
      | sbobj.Groups(8).Name = 'MotAgAandBFail1'
      | sbobj.Groups(8).Signals(1).Name = 'Call_Init1'
      | sbobj.Groups(8).Signals(1).XData = [0 10]
      | sbobj.Groups(8).Signals(1).YData = [0 0]
      | sbobj.Groups(8).Signals(2).Name = 'Call_Per1'
      | sbobj.Groups(8).Signals(2).XData = [0 0.002 0.002 10]
      | sbobj.Groups(8).Signals(2).YData = [1 1 0 0]
      | sbobj.Groups(8).Signals(3).Name = 'MotAgA'
      | sbobj.Groups(8).Signals(3).XData = [0 0.020202020202 0.040404040404 0.0606060606061 0.0808080808081 0.10101010101 0.121212121212 0.141414141414 0.161616161616 0.181818181818 0.20202020202 0.222222222222 ... (496 elements, 1x496)]
      | sbobj.Groups(8).Signals(3).YData = [0.5 0.531711959828 0.563296226787 0.59462562218 0.625573993591 0.656016722849 0.68583122783 0.714897456045 0.74309836805 0.770320408728 0.796453964527 0.821393804843 ... (496 elements, 1x496)]
      | sbobj.Groups(8).Signals(4).Name = 'MotAgAQlfr'
      | sbobj.Groups(8).Signals(4).XData = [0 0.305 1 1 3.005 3.005 10]
      | sbobj.Groups(8).Signals(4).YData = [1 1 1 2 1 2 2]
      | sbobj.Groups(8).Signals(5).Name = 'MotAgB'
      | sbobj.Groups(8).Signals(5).XData = [0 0.020202020202 0.040404040404 0.0606060606061 0.0808080808081 0.10101010101 0.121212121212 0.141414141414 0.161616161616 0.181818181818 0.20202020202 0.222222222222 ... (500 elements, 1x500)]
      | sbobj.Groups(8).Signals(5).YData = [0.5 0.531711959828 0.563296226787 0.59462562218 0.625573993591 0.656016722849 0.68583122783 0.714897456045 0.74309836805 0.770320408728 0.796453964527 0.821393804843 ... (500 elements, 1x500)]
      | sbobj.Groups(8).Signals(6).Name = 'FailRollingCounterB'
      | sbobj.Groups(8).Signals(6).XData = [0 0.5 10]
      | sbobj.Groups(8).Signals(6).YData = [0 0 0]
      | sbobj.Groups(8).Signals(7).Name = 'MotAgBQlfr'
      | sbobj.Groups(8).Signals(7).XData = [0 10]
      | sbobj.Groups(8).Signals(7).YData = [1 1]
  Call_Init1 : Outport  Tag=STV Outport
  Call_Per1 : Outport  Tag=STV Outport  Port=2
  MotAgA : Outport  Tag=STV Outport  Port=3
  MotAgAQlfr : Outport  Tag=STV Outport  Port=4
  MotAgB : Outport  Tag=STV Outport  Port=5
  FailRollingCounterB : Outport  Tag=STV Outport  Port=6
  MotAgBQlfr : Outport  Tag=STV Outport  Port=7
  wires:
  FromWs/1 -> Demux/1
  Demux/1 -> Call_Init1/1
  Demux/2 -> Call_Per1/1
  Demux/3 -> MotAgA/1
  Demux/4 -> MotAgAQlfr/1
  Demux/5 -> MotAgB/1
  Demux/6 -> FailRollingCounterB/1
  Demux/7 -> MotAgBQlfr/1

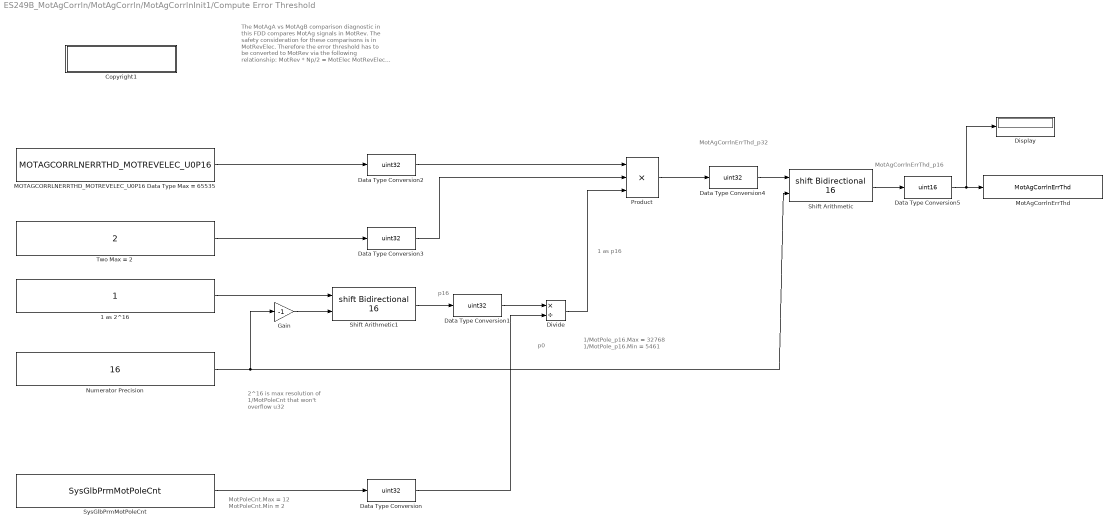
== system ES249B_MotAgCorrln/MotAgCorrln/MotAgCorrlnInit1/Compute Error Threshold ==
  note: MotAgCorrlnErrThd_p32
  note: p16
  note: p0
  note: 2^16 is max resolution
      | of 1/MotPoleCnt that won't
      | overflow u32
  note: MotPoleCnt.Max = 12
      | MotPoleCnt.Min = 2
  note: The MotAgA vs MotAgB comparison diagnostic
      | in this FDD compares MotAg signals in MotRev.
      | The safety consideration for these comparisons
      | is in MotRevElec.  Therefore the error threshold
      | has to be converted to MotRev via the following
      | relationship:
      |
      | MotRev * Np/2 = MotElec
      | MotRevElec * 2/Np = MotRev
  note: 1/MotPole_p16.Max = 32768
      | 1/MotPole_p16.Min = 5461
  note: 1 as p16
  note: MotAgCorrlnErrThd_p16
  1 as 2^16 : Constant  OutDataTypeStr=uint32
  Copyright1 : Subsystem  Description=|  RequirementInfo={} %GIDa_bacad073_da82_4802_ac19_55ca73cc7f3d  mask(Copyright Information){none=on}
      | Copyright info block.                                               
      |                                                                     
      | Place copyright information at the top of every subsystem in design.
      mask prompts: none "No parameters"
      mask help: Place copyright information at the top of every subsystem in design.
      mask Display:
      | NxtrConf = 'Nexteer Confidential';
      | 
      | sys = bdroot; %handle for the current model ("system")
      | first = get_param(sys,'Created');
      | if(isempty(first))
      |     first = datestr(now,'yyyy');
      | else
      |     first = first(end-3:end);  %year is last four digits
      | end
      | 
      | last = get_param(sys,'LastModifiedDate');
      | if isempty(last)
      |     last = datestr(now,'yyyy');
      | else
      |     last = last(end-3:end);
      | end
      | 
      | if strcmp(first,last)
      |     fprintf('%s\nCopyright  %s Nexteer',NxtrConf,first);
      | else
      |     fprintf('%s\n%s%s-%s Nexteer',NxtrConf,char(169),first,last);
      | end
  Data Type Conversion{,1..4} (5 alike) : DataTypeConversion  OutDataTypeStr=uint32
  Data Type Conversion5 : DataTypeConversion  OutDataTypeStr=uint16
  Display : Display
  Divide : Product  Inputs=*/
  Gain : Gain  Gain=-1  OutDataTypeStr=int8
  MOTAGCORRLNERRTHD_MOTREVELEC_U0P16 Data Type Max = 65535 : Constant  Value=MOTAGCORRLNERRTHD_MOTREVELEC_U0P16
  MotAgCorrlnErrThd : DataStoreWrite  DataStoreName=MotAgCorrlnErrThd
  Numerator Precision : Constant  Value=16  OutDataTypeStr=int8
  Product : Product  Inputs=3
  Shift Arithmetic : ArithShift  BitShiftNumberSource=Input port  BitShiftNumber=16
      settings: InputPortMap=u0,p1
  Shift Arithmetic1 : ArithShift  BitShiftNumberSource=Input port  BitShiftNumber=16
      settings: InputPortMap=u0,p1
  SysGlbPrmMotPoleCnt : Constant  Value=SysGlbPrmMotPoleCnt
  Two Max = 2 : Constant  Value=2  OutDataTypeStr=uint32
  wires:
  SysGlbPrmMotPoleCnt/1 -> Data Type Conversion/1
  1 as 2^16/1 -> Shift Arithmetic1/1
  Shift Arithmetic1/1 -> Data Type Conversion1/1
  Data Type Conversion/1 -> Divide/2
  MOTAGCORRLNERRTHD_MOTREVELEC_U0P16 Data Type Max = 65535/1 -> Data Type Conversion2/1
  Two Max = 2/1 -> Data Type Conversion3/1
  Divide/1 -> Product/3
  Product/1 -> Data Type Conversion4/1
  Data Type Conversion3/1 -> Product/2
  Data Type Conversion2/1 -> Product/1
  Data Type Conversion5/1 -> Display/1, MotAgCorrlnErrThd/1
  Data Type Conversion4/1 -> Shift Arithmetic/1
  Shift Arithmetic/1 -> Data Type Conversion5/1
  Numerator Precision/1 -> Gain/1, Shift Arithmetic/2
  Gain/1 -> Shift Arithmetic1/2
  Data Type Conversion1/1 -> Divide/1

== system ES249B_MotAgCorrln/MotAgCorrln/MotAgCorrlnInit1/Copyright1 ==

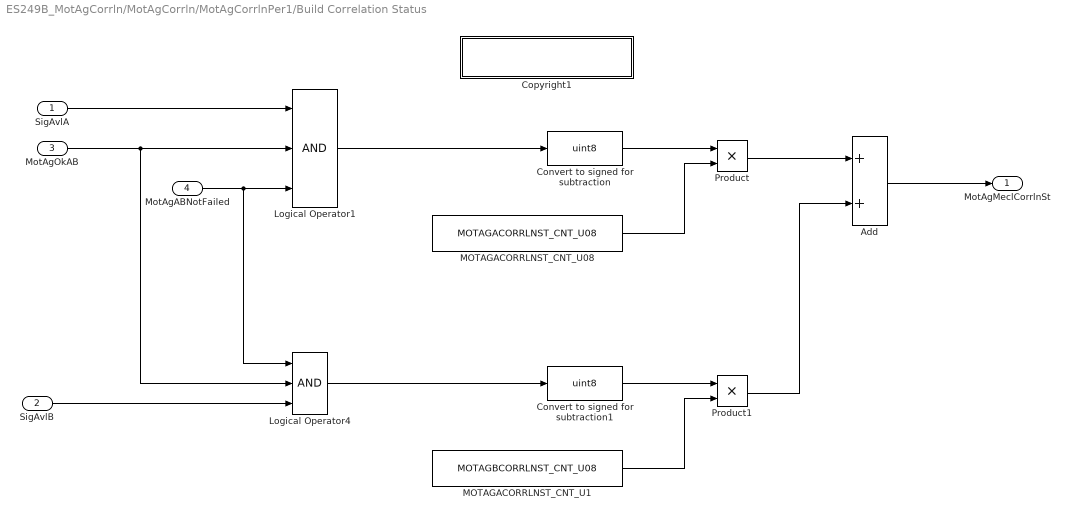
== system ES249B_MotAgCorrln/MotAgCorrln/MotAgCorrlnPer1/Build Correlation Status ==
  SigAvlA : Inport
  SigAvlB : Inport  Port=2
  MotAgOkAB : Inport  Port=3
  MotAgABNotFailed : Inport  Port=4
  Add : Sum
  Convert to signed for subtraction : DataTypeConversion  RequirementInfo={} %GIDa_3c43ff3c_738e_4afb_8a4c_067af10b302b  OutDataTypeStr=uint8
  Convert to signed for subtraction1 : DataTypeConversion  RequirementInfo={} %GIDa_b3174f25_a659_488f_90d8_daceb445e8d5  OutDataTypeStr=uint8
  Copyright1 : Subsystem  Description=|  RequirementInfo={} %GIDa_8df0f2c9_9123_4ed0_8405_91a2355391fa  mask(Copyright Information){none=on}
      | Copyright info block.                                               
      |                                                                     
      | Place copyright information at the top of every subsystem in design.
      mask prompts: none "No parameters"
      mask help: Place copyright information at the top of every subsystem in design.
      mask Display:
      | NxtrConf = 'Nexteer Confidential';
      | 
      | sys = bdroot; %handle for the current model ("system")
      | first = get_param(sys,'Created');
      | if(isempty(first))
      |     first = datestr(now,'yyyy');
      | else
      |     first = first(end-3:end);  %year is last four digits
      | end
      | 
      | last = get_param(sys,'LastModifiedDate');
      | if isempty(last)
      |     last = datestr(now,'yyyy');
      | else
      |     last = last(end-3:end);
      | end
      | 
      | if strcmp(first,last)
      |     fprintf('%s\nCopyright  %s Nexteer',NxtrConf,first);
      | else
      |     fprintf('%s\n%s%s-%s Nexteer',NxtrConf,char(169),first,last);
      | end
  Logical Operator1 : Logic  RequirementInfo={'linktype_rmi_doors' '0000cf69 (/E-STEER Core/SubSystem Specifications/Electrical Actuator/Control Module/FDD Module Requirements/EA4/ES249B_MotAgCorrln)' '#ES249B_91' 'true' 'REQ: ES249B_91' '' } %GIDa_dd4fdede_bbc5_41a2_9fe1_016ced5ebd43  Inputs=3  AllPortsSameDT=off  OutDataTypeStr=boolean
  Logical Operator4 : Logic  RequirementInfo={'linktype_rmi_doors' '0000cf69 (/E-STEER Core/SubSystem Specifications/Electrical Actuator/Control Module/FDD Module Requirements/EA4/ES249B_MotAgCorrln)' '#ES249B_93' 'true' 'REQ: ES249B_93' '' } %GIDa_ebb81955_3cd8_48a8_afb1_b1a311d2c14a  Inputs=3  AllPortsSameDT=off  OutDataTypeStr=boolean
  MOTAGACORRLNST_CNT_U08 : Constant  Value=MOTAGACORRLNST_CNT_U08
  MOTAGACORRLNST_CNT_U1 : Constant  Value=MOTAGBCORRLNST_CNT_U08
  Product : Product
  Product1 : Product
  MotAgMeclCorrlnSt : Outport
  wires:
  Logical Operator1/1 -> Convert to signed for subtraction/1
  Convert to signed for subtraction/1 -> Product/1
  MOTAGACORRLNST_CNT_U08/1 -> Product/2
  Logical Operator4/1 -> Convert to signed for subtraction1/1
  Convert to signed for subtraction1/1 -> Product1/1
  MOTAGACORRLNST_CNT_U1/1 -> Product1/2
  Product/1 -> Add/1
  Product1/1 -> Add/2
  Add/1 -> MotAgMeclCorrlnSt/1
  SigAvlA/1 -> Logical Operator1/1
  SigAvlB/1 -> Logical Operator4/3
  MotAgOkAB/1 -> Logical Operator4/2, Logical Operator1/2
  MotAgABNotFailed/1 -> Logical Operator4/1, Logical Operator1/3

== system ES249B_MotAgCorrln/MotAgCorrln/MotAgCorrlnPer1/Copyright1 ==

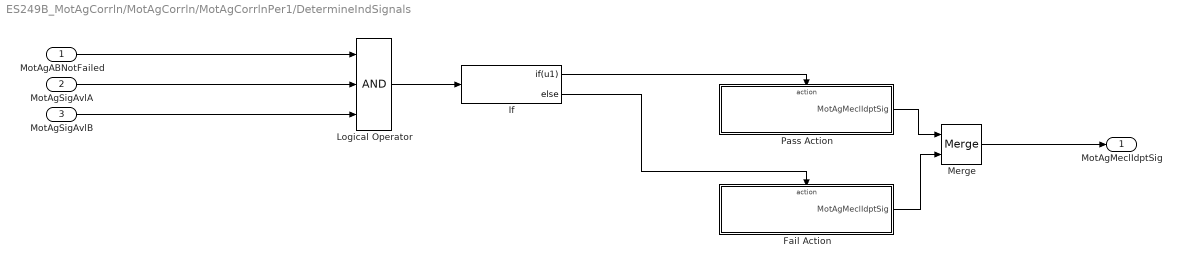
== system ES249B_MotAgCorrln/MotAgCorrln/MotAgCorrlnPer1/DetermineIndSignals ==
  MotAgABNotFailed : Inport
  MotAgSigAvlA : Inport  Port=2
  MotAgSigAvlB : Inport  Port=3
  "Fail Action " : Subsystem  RequirementInfo={'linktype_rmi_doors' '0000cf69 (/E-STEER Core/SubSystem Specifications/Electrical Actuator/Control Module/FDD Module Requirements/EA4/ES249B_MotAgCorrln)' '#ES249B_101' 'true' 'REQ: ES249B_101' '' } %GIDa_5ca1e778_167b_457c_8759_54104e67914e  TreatAsAtomicUnit=on
  If : If  RequirementInfo={} %GIDa_02665ea6_e505_44a1_82d9_89c581a4a628  IfExpression=u1
  Logical Operator : Logic  RequirementInfo={'linktype_rmi_doors' '0000cf69 (/E-STEER Core/SubSystem Specifications/Electrical Actuator/Control Module/FDD Module Requirements/EA4/ES249B_MotAgCorrln)' '#ES249B_96' 'true' 'REQ: ES249B_96' '' ; 'linktype_rmi_doors' '0000cf69 (/E-STEER Core/SubSystem Specifications/Electrical Actuator/Control Module/FDD Module Requirements/EA4/ES249B_MotAgCorrln)' '#ES249B_101' 'true' 'REQ: ES249B_101' '' } %GIDa_f8baa016_c99a_492c_81fc_e6cb7294f61a  Inputs=3  AllPortsSameDT=off  OutDataTypeStr=boolean
  Merge : Merge
  "Pass Action " : Subsystem  RequirementInfo={'linktype_rmi_doors' '0000cf69 (/E-STEER Core/SubSystem Specifications/Electrical Actuator/Control Module/FDD Module Requirements/EA4/ES249B_MotAgCorrln)' '#ES249B_96' 'true' 'REQ: ES249B_96' '' } %GIDa_ebd042ce_1372_4b27_915f_9944f04a3100  TreatAsAtomicUnit=on
  MotAgMeclIdptSig : Outport
  wires:
  MotAgSigAvlB/1 -> Logical Operator/3
  If/2 -> "Fail Action "/Action
  Merge/1 -> MotAgMeclIdptSig/1
  "Pass Action "/1(MotAgMeclIdptSig) -> Merge/1
  "Fail Action "/1(MotAgMeclIdptSig) -> Merge/2
  Logical Operator/1 -> If/1
  If/1 -> "Pass Action "/Action
  MotAgSigAvlA/1 -> Logical Operator/2
  MotAgABNotFailed/1 -> Logical Operator/1

== system ES249B_MotAgCorrln/MotAgCorrln/MotAgCorrlnPer1/FltInj_u08  ==
  note: This block requires no modification by FDD author.
      |
      | This block does not actually simulate any fault injection.  It is simply a pass-thru.
      |
      | The Constant port (#2) simply terminates its signal, but we are trying to force the FDD author
      | to properly use the FltInjectionLocType enumeration in FDD model.
  note: EA4.x Fault Injection
  Signal_In : Inport
  Constant : Inport  Port=2
  Copyright1 : Subsystem  Description=|  RequirementInfo={} %GIDa_0eace49f_b789_449d_b1ad_5a467ed07a04  mask(Copyright Information){none=on}
      | Copyright info block.                                               
      |                                                                     
      | Place copyright information at the top of every subsystem in design.
      mask prompts: none "No parameters"
      mask help: Place copyright information at the top of every subsystem in design.
      mask Display:
      | NxtrConf = 'Nexteer Confidential';
      | 
      | sys = bdroot; %handle for the current model ("system")
      | first = get_param(sys,'Created');
      | if(isempty(first))
      |     first = datestr(now,'yyyy');
      | else
      |     first = first(end-3:end);  %year is last four digits
      | end
      | 
      | last = get_param(sys,'LastModifiedDate');
      | if isempty(last)
      |     last = datestr(now,'yyyy');
      | else
      |     last = last(end-3:end);
      | end
      | 
      | if strcmp(first,last)
      |     fprintf('%s\nCopyright  %s Nexteer',NxtrConf,first);
      | else
      |     fprintf('%s\n%s%s-%s Nexteer',NxtrConf,char(169),first,last);
      | end
  Terminator : Terminator
  Signal_Out : Outport
  wires:
  Signal_In/1 -> Signal_Out/1
  Constant/1 -> Terminator/1

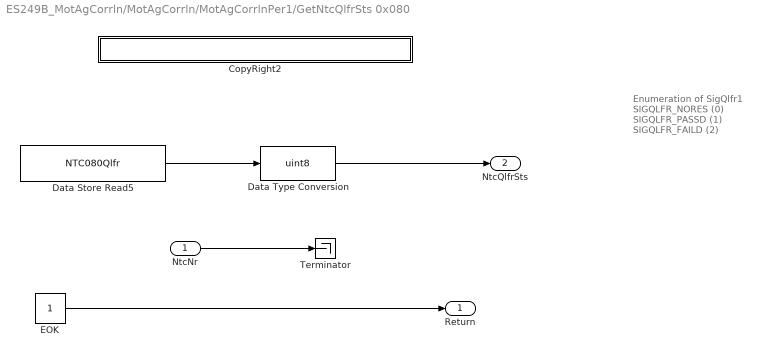
== system ES249B_MotAgCorrln/MotAgCorrln/MotAgCorrlnPer1/GetNtcQlfrSts 0x080  ==
  note: Enumeration of SigQlfr1
      |         SIGQLFR_NORES   (0)
      |         SIGQLFR_PASSD    (1)
      |         SIGQLFR_FAILD      (2)
  NtcNr : Inport
  CopyRight2 : Subsystem  Description=|  mask(Copyright Information){none=on}
      | Copyright info block.                                               
      |                                                                     
      | Place copyright information at the top of every subsystem in design.
      mask prompts: none "No parameters"
      mask help: Place copyright information at the top of every subsystem in design.
      mask Display:
      | NxtrConf = 'Nexteer Confidential';
      | 
      | sys = bdroot; %handle for the current model ("system")
      | first = get_param(sys,'Created');
      | first = first(end-3:end);  %year is last four digits
      | 
      | last = get_param(sys,'LastModifiedDate');
      | if isempty(last)
      |     last = datestr(now,'yyyy');
      | else
      |     last = last(end-3:end);
      | end
      | 
      | if strcmp(first,last)
      |     fprintf('%s -- Copyright %s Nexteer',NxtrConf,first)
      | else
      |     fprintf('%s -- %s%s- %s Nexteer',NxtrConf,char(169),first,last)
      | end
  Data Store Read5 : DataStoreRead  DataStoreName=NTC080Qlfr
  Data Type Conversion : DataTypeConversion  OutDataTypeStr=uint8
  EOK : Constant  OutDataTypeStr=uint8
  Terminator : Terminator
  Return : Outport  InitialOutput=1
  NtcQlfrSts : Outport  Port=2
  wires:
  Data Store Read5/1 -> Data Type Conversion/1
  EOK/1 -> Return/1
  NtcNr/1 -> Terminator/1
  Data Type Conversion/1 -> NtcQlfrSts/1

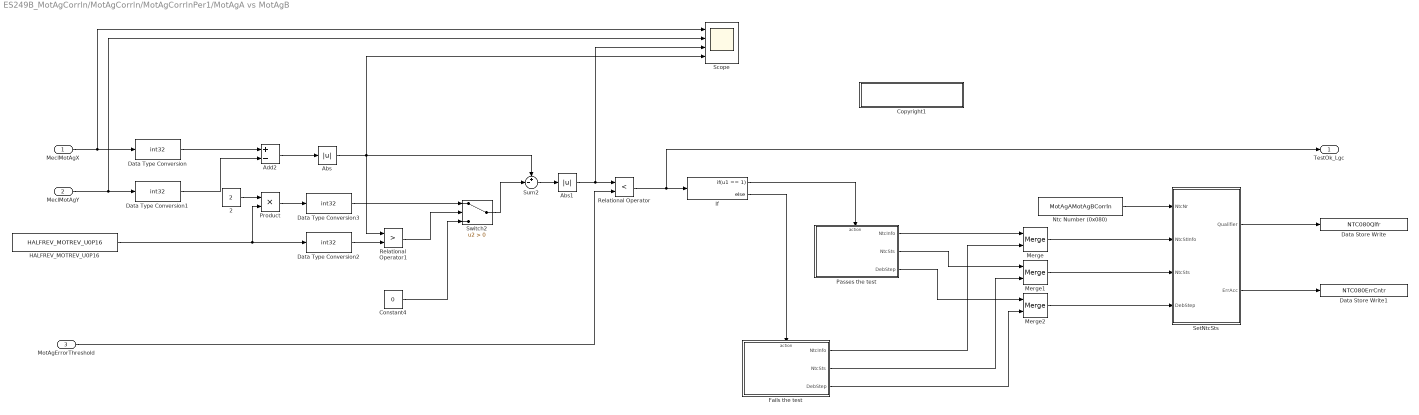
== system ES249B_MotAgCorrln/MotAgCorrln/MotAgCorrlnPer1/MotAgA vs MotAgB ==
  MeclMotAgX : Inport  RequirementInfo={} %GIDa_209a8ec2_f83a_4596_ac14_016e97e43532
  MeclMotAgY : Inport  RequirementInfo={} %GIDa_3879b633_065b_44db_a611_7209c5040c41  Port=2
  MotAgErrorThreshold : Inport  RequirementInfo={} %GIDa_52fd4367_99f4_419f_a569_0cba8f97a327  Port=3
  2 : Constant  Value=2  OutDataTypeStr=int32
  Abs : Abs
  Abs1 : Abs
  Add2 : Sum  RequirementInfo={'linktype_rmi_doors' '0000cf69 (/E-STEER Core/SubSystem Specifications/Electrical Actuator/Control Module/FDD Module Requirements/EA4/ES249B_MotAgCorrln)' '#ES249B_28' 'true' 'REQ: ES249B_28' '' } %GIDa_89d79b4a_b8b1_46bd_92a0_8fa9f55b18cb  Inputs=+-  AccumDataTypeStr=int32
  Constant4 : Constant  Value=0  OutDataTypeStr=int32
  Copyright1 : Subsystem  Description=|  RequirementInfo={} %GIDa_43863c04_fa5e_452c_a1b7_4fa30e8bd61b  mask(Copyright Information){none=on}
      | Copyright info block.                                               
      |                                                                     
      | Place copyright information at the top of every subsystem in design.
      mask prompts: none "No parameters"
      mask help: Place copyright information at the top of every subsystem in design.
      mask Display:
      | NxtrConf = 'Nexteer Confidential';
      | 
      | sys = bdroot; %handle for the current model ("system")
      | first = get_param(sys,'Created');
      | if(isempty(first))
      |     first = datestr(now,'yyyy');
      | else
      |     first = first(end-3:end);  %year is last four digits
      | end
      | 
      | last = get_param(sys,'LastModifiedDate');
      | if isempty(last)
      |     last = datestr(now,'yyyy');
      | else
      |     last = last(end-3:end);
      | end
      | 
      | if strcmp(first,last)
      |     fprintf('%s\nCopyright  %s Nexteer',NxtrConf,first);
      | else
      |     fprintf('%s\n%s%s-%s Nexteer',NxtrConf,char(169),first,last);
      | end
  Data Store Write : DataStoreWrite  RequirementInfo={} %GIDa_9512697d_c087_4109_9134_0a84db0896e8  DataStoreName=NTC080Qlfr
  Data Store Write1 : DataStoreWrite  RequirementInfo={} %GIDa_09fa0ad2_fadc_4e01_82b6_87880c397f4c  DataStoreName=NTC080ErrCntr
  Data Type Conversion{,1..3} (4 alike) : DataTypeConversion  OutDataTypeStr=int32
  Fails the test : Subsystem  RequirementInfo={'linktype_rmi_doors' '0000cf69 (/E-STEER Core/SubSystem Specifications/Electrical Actuator/Control Module/FDD Module Requirements/EA4/ES249B_MotAgCorrln)' '#ES249B_28' 'true' 'REQ: ES249B_28' '' } %GIDa_32330a11_135a_4d4a_b6a9_5738b4884140  TreatAsAtomicUnit=on
  HALFREV_MOTREV_U0P16 : Constant  Value=HALFREV_MOTREV_U0P16  OutDataTypeStr=int32
  If : If  RequirementInfo={} %GIDa_4a7e1530_6c57_410a_8590_40bd88f14402  IfExpression=u1 == 1
  Merge : Merge  RequirementInfo={} %GIDa_5c5d4849_b0d7_417e_8e37_be493b9884db
  Merge1 : Merge  RequirementInfo={} %GIDa_96dc7a19_089f_4a81_91dd_98b954b09d33
  Merge2 : Merge  RequirementInfo={} %GIDa_445cf7d9_fe34_4f83_8f83_84d725eb67cd
  Ntc Number (0x080) : Constant  RequirementInfo={} %GIDa_17484570_857f_4649_8079_9998f179e352  Value=MotAgAMotAgBCorrln
  Passes the test : Subsystem  RequirementInfo={'linktype_rmi_doors' '0000cf69 (/E-STEER Core/SubSystem Specifications/Electrical Actuator/Control Module/FDD Module Requirements/EA4/ES249B_MotAgCorrln)' '#ES249B_31' 'true' 'REQ: ES249B_31' '' } %GIDa_2e2aa5eb_d2a7_4382_b0d6_a86d4a99b386  TreatAsAtomicUnit=on
  Product : Product
  Relational Operator : RelationalOperator  RequirementInfo={} %GIDa_e81e555f_20f9_4e1d_8333_9ac819d3840d  Operator=<  OutDataTypeStr=boolean
  Relational Operator1 : RelationalOperator  RequirementInfo={'linktype_rmi_doors' '0000cf69 (/E-STEER Core/SubSystem Specifications/Electrical Actuator/Control Module/FDD Module Requirements/EA4/ES249B_MotAgCorrln)' '#ES249B_107' 'true' 'REQ: ES249B_107' '' } %GIDa_f4cbc6ad_5b9b_451e_95d2_df775aceae4b  Operator=>  OutDataTypeStr=boolean
  Scope : Scope  NumInputPorts=4
      settings: TimeRange=1  YMin=0~-5~-5~-5  YMax=8~5~5~5
  SetNtcSts : Subsystem  RequirementInfo={'linktype_rmi_doors' '0000cf69 (/E-STEER Core/SubSystem Specifications/Electrical Actuator/Control Module/FDD Module Requirements/EA4/ES249B_MotAgCorrln)' '#ES249B_22' 'true' 'REQ: ES249B_22' '' } %GIDa_372e5e5c_ac16_4961_ac82_62e12ce3987b  TreatAsAtomicUnit=on
      settings: RTWSystemCode=Inline
  Sum2 : Sum  Inputs=+-|
  Switch2 : Switch  Criteria=u2 > Threshold
  TestOk_Lgc : Outport  RequirementInfo={} %GIDa_58faf550_67b9_443b_9b7a_437f5011a6c4
  wires:
  Relational Operator/1 -> If/1, TestOk_Lgc/1
  If/1 -> Passes the test/Action
  If/2 -> Fails the test/Action
  Ntc Number (0x080)/1 -> SetNtcSts/1(NtcNr)
  Merge/1 -> SetNtcSts/2(NtcStInfo)
  Merge1/1 -> SetNtcSts/3(NtcSts)
  Merge2/1 -> SetNtcSts/4(DebStep)
  Passes the test/1(NtcInfo) -> Merge/1
  Fails the test/1(NtcInfo) -> Merge/2
  Passes the test/2(NtcSts) -> Merge1/1
  Fails the test/2(NtcSts) -> Merge1/2
  Fails the test/3(DebStep) -> Merge2/2
  Passes the test/3(DebStep) -> Merge2/1
  SetNtcSts/1(Qualifier) -> Data Store Write/1
  SetNtcSts/2(ErrAcc) -> Data Store Write1/1
  Abs1/1 -> Scope/3, Relational Operator/1
  MotAgErrorThreshold/1 -> Relational Operator/2
  Data Type Conversion/1 -> Add2/1
  Sum2/1 -> Abs1/1
  Data Type Conversion1/1 -> Add2/2
  Switch2/1 -> Sum2/2
  Constant4/1 -> Switch2/3
  Relational Operator1/1 -> Switch2/2
  HALFREV_MOTREV_U0P16/1 -> Product/2, Data Type Conversion2/1
  Abs/1 -> Scope/4, Sum2/1, Relational Operator1/1
  Add2/1 -> Abs/1
  MeclMotAgX/1 -> Scope/1, Data Type Conversion/1
  MeclMotAgY/1 -> Scope/2, Data Type Conversion1/1
  Data Type Conversion2/1 -> Relational Operator1/2
  2/1 -> Product/1
  Product/1 -> Data Type Conversion3/1
  Data Type Conversion3/1 -> Switch2/1

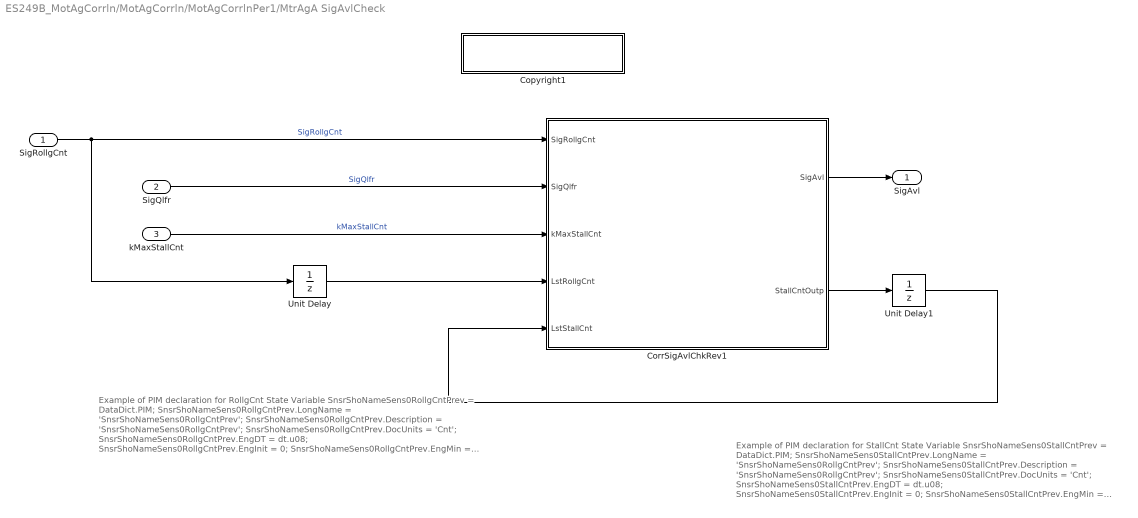
== system ES249B_MotAgCorrln/MotAgCorrln/MotAgCorrlnPer1/MtrAgA SigAvlCheck ==
  note: Example of PIM declaration for StallCnt State Variable
      |
      | SnsrShoNameSens0StallCntPrev = DataDict.PIM;
      | SnsrShoNameSens0StallCntPrev.LongName = 'SnsrShoNameSens0RollgCntPrev';
      | SnsrShoNameSens0StallCntPrev.Description = 'SnsrShoNameSens0RollgCntPrev';
      | SnsrShoNameSens0StallCntPrev.DocUnits = 'Cnt';
      | SnsrShoNameSens0StallCntPrev.EngDT = dt.u08;
      | SnsrShoNameSens0StallCntPrev.EngInit = 0;
      | SnsrShoNameSens0StallCntPrev.EngMin = 0;
      | SnsrShoNameSens0StallCntPrev.EngMax = 255;
      |
      |
      | *********  Need different state variable for each instance of this  subsystem ********
  note: Example of PIM declaration for RollgCnt State Variable
      |
      | SnsrShoNameSens0RollgCntPrev = DataDict.PIM;
      | SnsrShoNameSens0RollgCntPrev.LongName = 'SnsrShoNameSens0RollgCntPrev';
      | SnsrShoNameSens0RollgCntPrev.Description = 'SnsrShoNameSens0RollgCntPrev';
      | SnsrShoNameSens0RollgCntPrev.DocUnits = 'Cnt';
      | SnsrShoNameSens0RollgCntPrev.EngDT = dt.u08;
      | SnsrShoNameSens0RollgCntPrev.EngInit = 0;
      | SnsrShoNameSens0RollgCntPrev.EngMin = 0;
      | SnsrShoNameSens0RollgCntPrev.EngMax = 255;
      |
      |
      | *********  Need different state variable for each instance of this  subsystem ********
  SigRollgCnt : Inport  OutDataTypeStr=uint8
  SigQlfr : Inport  Port=2  OutDataTypeStr=uint8
  kMaxStallCnt : Inport  Port=3  OutDataTypeStr=uint8
  Copyright1 : Subsystem  Description=|  RequirementInfo={} %GIDa_9c9c1667_19aa_4844_bfe7_7465a4e2bb9e  mask(Copyright Information){none=on}
      | Copyright info block.                                               
      |                                                                     
      | Place copyright information at the top of every subsystem in design.
      mask prompts: none "No parameters"
      mask help: Place copyright information at the top of every subsystem in design.
      mask Display:
      | NxtrConf = 'Nexteer Confidential';
      | 
      | sys = bdroot; %handle for the current model ("system")
      | first = get_param(sys,'Created');
      | if(isempty(first))
      |     first = datestr(now,'yyyy');
      | else
      |     first = first(end-3:end);  %year is last four digits
      | end
      | 
      | last = get_param(sys,'LastModifiedDate');
      | if isempty(last)
      |     last = datestr(now,'yyyy');
      | else
      |     last = last(end-3:end);
      | end
      | 
      | if strcmp(first,last)
      |     fprintf('%s\nCopyright  %s Nexteer',NxtrConf,first);
      | else
      |     fprintf('%s\n%s%s-%s Nexteer',NxtrConf,char(169),first,last);
      | end
  CorrSigAvlChkRev1 : Stateflow chart  TreatAsAtomicUnit=on
  Unit Delay : UnitDelay  SampleTime=-1  StateName=MotAgCorrlnMotAgARollgCntPrev  StateMustResolveToSignalObject=on
      settings: AttributesFormatString=|
      | State Variable:
      | %<StateName>
  Unit Delay1 : UnitDelay  SampleTime=-1  StateName=MotAgCorrlnMotAgAStallCntPrev  StateMustResolveToSignalObject=on
      settings: AttributesFormatString=|
      | State Variable:
      | %<StateName>
  SigAvl : Outport
  wires:
  SigRollgCnt/1 -> Unit Delay/1, CorrSigAvlChkRev1/1(SigRollgCnt)  "SigRollgCnt"
  SigQlfr/1 -> CorrSigAvlChkRev1/2(SigQlfr)  "SigQlfr"
  kMaxStallCnt/1 -> CorrSigAvlChkRev1/3(kMaxStallCnt)  "kMaxStallCnt"
  Unit Delay/1 -> CorrSigAvlChkRev1/4(LstRollgCnt)
  CorrSigAvlChkRev1/2(StallCntOutp) -> Unit Delay1/1
  Unit Delay1/1 -> CorrSigAvlChkRev1/5(LstStallCnt)
  CorrSigAvlChkRev1/1(SigAvl) -> SigAvl/1
